simulink model "logicOperation"  (R2023b)
settings: Solver=VariableStepAuto  StartTime=0.0  StopTime=10.0  RelTol=1e-3
libraries: simulink x2
settings Model: Creator=NITRO  LastModifiedBy=NITRO

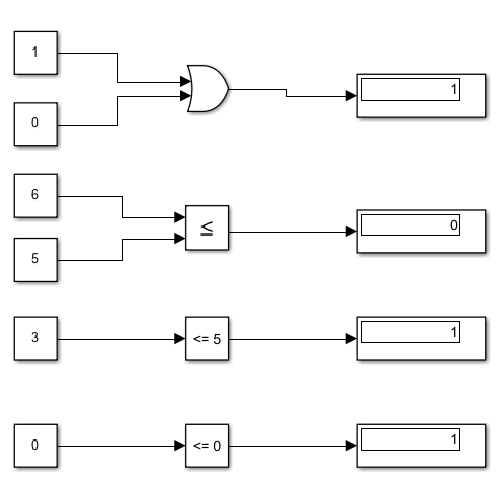
[thumbnail: Simulink's stored preview of the top-level diagram]
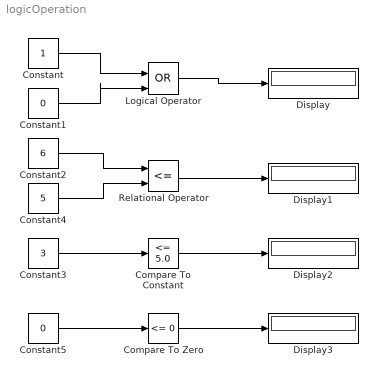
== system logicOperation ==
  Compare To Constant : simulink/Logic and Bit Operations/Compare To Constant  relop=<=  const=5.0  OutDataTypeStr=boolean
  Compare To Zero : simulink/Logic and Bit Operations/Compare To Zero  relop=<=  OutDataTypeStr=boolean
  Constant : Constant
  Constant1 : Constant  Value=0
  Constant2 : Constant  Value=6
  Constant3 : Constant  Value=3
  Constant4 : Constant  Value=5
  Constant5 : Constant  Value=0
  Display{,1..3} (4 alike) : Display
  Logical Operator : Logic  Operator=OR  IconShape=distinctive  AllPortsSameDT=off  OutDataTypeStr=boolean
  Relational Operator : RelationalOperator  Operator=<=  OutDataTypeStr=boolean  RndMeth=Simplest  InputSameDT=off
  wires:
  Compare To Zero/1 -> Display3/1
  Constant5/1 -> Compare To Zero/1
  Constant3/1 -> Compare To Constant/1
  Compare To Constant/1 -> Display2/1
  Relational Operator/1 -> Display1/1
  Logical Operator/1 -> Display/1
  Constant/1 -> Logical Operator/1
  Constant1/1 -> Logical Operator/2
  Constant2/1 -> Relational Operator/1
  Constant4/1 -> Relational Operator/2
